simulink model "ather_450x"  (R2021a)
settings: Solver=VariableStepAuto  StartTime=0  StopTime=2474  RelTol=1e-3
libraries: simulink_extras x1, autolibshared x1
settings Model: Creator=hp  LastModifiedBy=hp

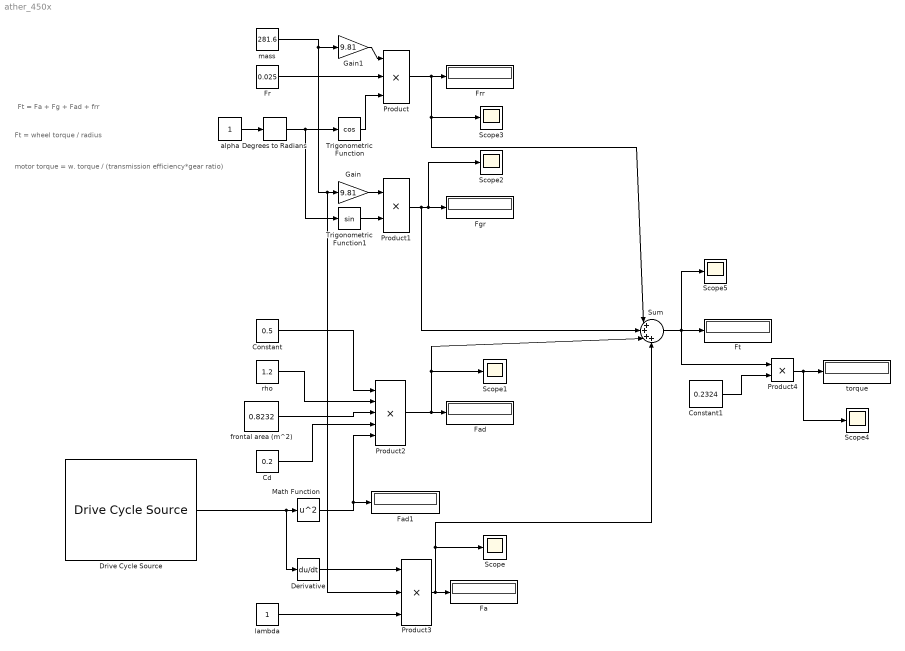
== system ather_450x ==
  note: motor torque = w. torque / (transmission efficiency*gear ratio)
  note: Ft = wheel torque / radius
  note: Ft = Fa + Fg + Fad + frr
  Cd : Constant  Value=0.2
  Constant : Constant  Value=0.5
  Constant1 : Constant  Value=0.2324
  Degrees to Radians : simulink_extras/Transformations/Degrees to Radians
  Derivative : Derivative
  Drive Cycle Source : autolibshared/Drive Cycle Source  cycleVar=FTP75  fileVar=cycleFTP75.mat  tfinal="2474  seconds"  cycleRepeat=off  outAccPort=off  outGearPort=off  gearList=No gear data  t_wot1=5  xdot_woto=0  xdot_wot1=30  t_wot2=20  xdot_wot2=0  t_wotend=30  srcUnit=m/s  outUnit=m/s  srcAccUnit=m/s/s  outAccUnit=m/s^2  dt=0  aMode=1  faultOption=off  velBnd=2  velBndUnit=mph  inUnit=m/s  timeBnd=1  failOption=off  stopSim=off  maxFaultCnt=10  maxFaultTime=2  maxTotFaultTime=15  traceOption=off  dtTrace=1  traceWindow=10  lastDCname=FTP75  lastOutUnit=mph  lastDT=0  lastTB=1  lastSB=2  forceCalcBound=off
      settings: SourceProductBaseCode=PW,DR,MT,UV,VE
  Fa : Display
  Fad : Display
  Fad1 : Display
  Fgr : Display
  Fr : Constant  Value=0.025
  Frr : Display
  Ft : Display
  Gain : Gain  Gain=9.81
  Gain1 : Gain  Gain=9.81
  Math Function : Math  Operator=square  SaturateOnIntegerOverflow=on
  Product : Product  Inputs=3
  Product1 : Product
  Product2 : Product  Inputs=5
  Product3 : Product  Inputs=3
  Product4 : Product
  Scope{,1..5} (6 alike) : Scope
  Sum : Sum  Inputs=|++++
  Trigonometric Function : Trigonometry  Operator=cos
  Trigonometric Function1 : Trigonometry
  alpha : Constant
  frontal area (m^2) : Constant  Value=0.8232
  lambda : Constant
  mass : Constant  Value=281.6
  rho : Constant  Value=1.2
  torque : Display
  wires:
  alpha/1 -> Degrees to Radians/1
  Product/1 -> Scope3/1, Sum/1, Frr/1
  Product1/1 -> Sum/2, Scope2/1, Fgr/1
  Degrees to Radians/1 -> Trigonometric Function/1, Trigonometric Function1/1
  Trigonometric Function/1 -> Product/3
  Fr/1 -> Product/2
  Trigonometric Function1/1 -> Product1/2
  Drive Cycle Source/1 -> Derivative/1, Math Function/1
  frontal area (m^2)/1 -> Product2/3
  rho/1 -> Product2/2
  Constant/1 -> Product2/1
  Cd/1 -> Product2/4
  Math Function/1 -> Fad1/1, Product2/5
  Product2/1 -> Sum/3, Scope1/1, Fad/1
  mass/1 -> Gain/1, Product3/2, Gain1/1
  lambda/1 -> Product3/3
  Product3/1 -> Scope/1, Sum/4, Fa/1
  Derivative/1 -> Product3/1
  Sum/1 -> Scope5/1, Product4/1, Ft/1
  Product4/1 -> Scope4/1, torque/1
  Constant1/1 -> Product4/2
  Gain/1 -> Product1/1
  Gain1/1 -> Product/1
